simulink model "rocket_upwork"  (R2026a)
settings: Solver=ode15s  StopTime=150  FixedStep=1/3000  MaxStep=0.001  RelTol=1e-6
InitFcn:
  | matl;
undefined symbols (not defined in the file or in its folder): rocket
libraries: aerolibasang x2, simulink x1, aerolibfltsims x1, aerolibatmos2 x1, aerolibadyn x1
settings Model: Creator=evilcatzilla  LastModifiedBy=carlos
settings SolverCC: MaxConsecutiveMinStep=10  SolverResetMethod=Robust
settings SimscapeCC: SimscapeLogDataHistory=5000  SimscapeLogType=none  SimscapeNominalValues="[{\"value\":\"1\",\"unit\":\"A\"},{\"value\":\"1\",\"unit\":\"bar\"},{\"value\":\"1\",\"unit\":\"cm^2\"},{\"value\":\"1\",\"unit\":\"cm^3/s\"},{\"value\":\"1\",\"unit\":\"kJ/kg\"},{\"value\":\"1\",\"unit\":\"kW\"},{\"value\":\"1\",\"unit\":\"l\"},{\"value\":\"1\",\"unit\":\"N\"},{\"value\":\"1\",\"unit\":\"N*m\"},{\"value\":\"1\",\"unit\":\"V\"}]"  SimscapeLogDecimation=1

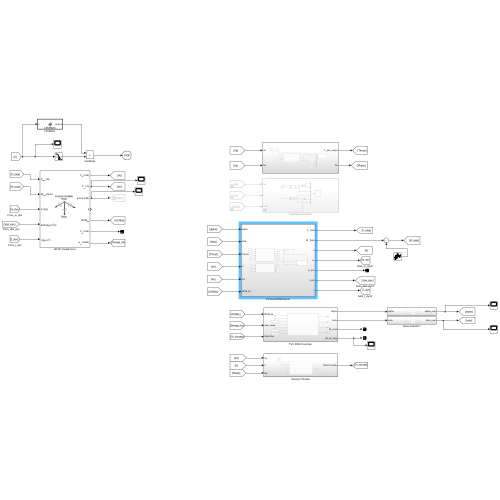
[thumbnail: Simulink's stored preview of the top-level diagram]
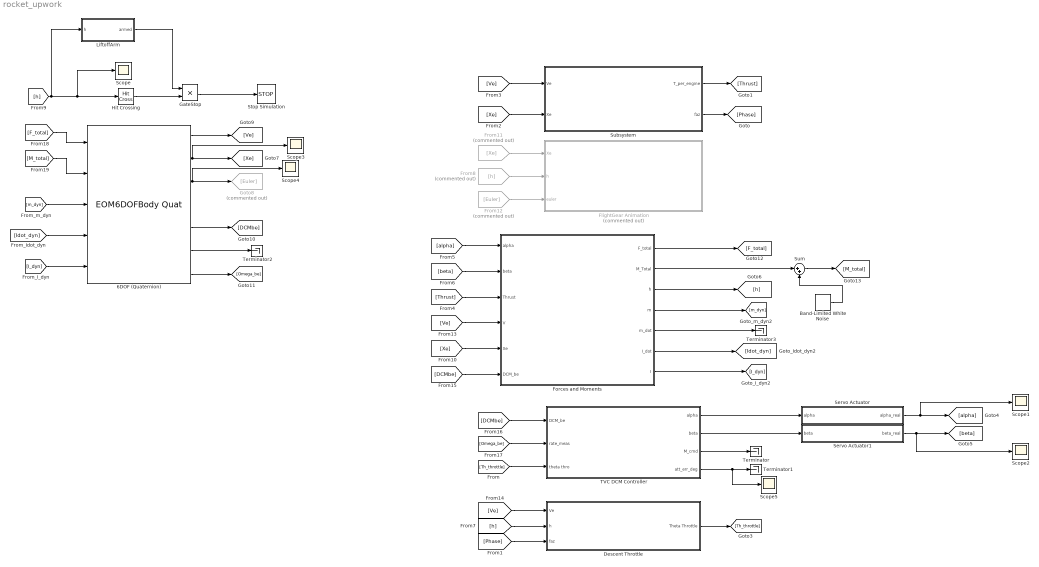
== system rocket_upwork ==
  6DOF (Quaternion) : EOM6DOFBodyQuat  mtype=Custom Variable  eul_0=[0 deg2rad(85) 0]  mass_0=rocket.m0_computed  mass_f=2.0  inertia=diag([rocket.Ixx, rocket.Iyy, rocket.Izz])
  Band-Limited White Noise : simulink/Sources/Band-Limited White Noise  Cov=4e-6  Ts=0.01  seed=[23341 23342 23343]
  Descent Throttle : Subsystem
  FlightGear Animation : Subsystem  Commented=on
  Forces and Moments : Subsystem
  From11 : From  Commented=on  GotoTag=Xe
  From12 : From  Commented=on  GotoTag=Euler
  From8 : From  Commented=on  GotoTag=h
  GateStop : Product
  Goto8 : Goto  Commented=on  GotoTag=Euler
  Hit Crossing : HitCross  HitCrossingDirection=falling
  LiftoffArm : MATLAB Function  TreatAsAtomicUnit=on  SystemSampleTime=0.001
  Scope{,1..5} (6 alike) : Scope
      Scope settings: ActiveDisplayYMinimum=-1.94208  ActiveDisplayYMaximum=17.47869
      Scope1 settings: ActiveDisplayYMinimum=-0.94567  ActiveDisplayYMaximum=1.34881  DataLoggingVariableName=ScopeData2
      Scope2 settings: ActiveDisplayYMinimum=-1.10174  ActiveDisplayYMaximum=1.06476  DataLoggingVariableName=ScopeData3
      Scope3 settings: ActiveDisplayYMinimum=-25.2743  ActiveDisplayYMaximum=72.10268  DataLoggingVariableName=ScopeData4
      Scope4 settings: ActiveDisplayYMinimum=-3.9266  ActiveDisplayYMaximum=3.92558  DataLoggingVariableName=ScopeData5
      Scope5 settings: ActiveDisplayYMinimum=-20.36974  ActiveDisplayYMaximum=7.70273  DataLoggingVariableName=ScopeData7
  Servo Actuator : Subsystem
  Servo Actuator1 : Subsystem
  Stop Simulation : Stop
  Subsystem : Subsystem
  Sum : Sum  Inputs=|++
  TVC DCM Controller : Subsystem
  Terminator{,1..3} (4 alike) : Terminator
  wires:
  TVC DCM Controller/3(M_cmd) -> Terminator/1
  TVC DCM Controller/4(att_err_deg) -> Terminator1/1, Scope5/1
  [h] -> Descent Throttle/2(h)
  From8/1 -> FlightGear Animation/2(h)
  From11/1 -> FlightGear Animation/1(Xe)
  From12/1 -> FlightGear Animation/3(euler)
  [Ve] -> Descent Throttle/1(Ve)
  [DCMbe] -> TVC DCM Controller/1(DCM_be)
  [Omega_be] -> TVC DCM Controller/2(rate_meas)
  Band-Limited White Noise/1 -> Sum/2
  Sum/1 -> [M_total]
  TVC DCM Controller/1(alpha) -> Servo Actuator/1(alpha)
  Servo Actuator/1(alpha_real) -> [alpha], Scope1/1
  TVC DCM Controller/2(beta) -> Servo Actuator1/1(beta)
  Servo Actuator1/1(beta_real) -> [beta], Scope2/1
  Descent Throttle/1(Theta Throttle) -> [Th_throttle]
  [Th_throttle] -> TVC DCM Controller/3(theta thro)
  [Phase] -> Descent Throttle/3(faz)
  Subsystem/2(faz) -> [Phase]
  Subsystem/1(T_per_engine) -> [Thrust]
  [Xe] -> Subsystem/2(Xe)
  [Ve] -> Subsystem/1(Ve)
  [I_dyn] -> 6DOF (Quaternion)/5
  [Idot_dyn] -> 6DOF (Quaternion)/4
  [m_dyn] -> 6DOF (Quaternion)/3
  [F_total] -> 6DOF (Quaternion)/1
  [M_total] -> 6DOF (Quaternion)/2
  [h] -> Scope/1, Hit Crossing/1, LiftoffArm/1(h)
  Forces and Moments/7(I) -> [I_dyn]
  Forces and Moments/6(I_dot) -> [Idot_dyn]
  Forces and Moments/5(m_dot) -> Terminator3/1
  Forces and Moments/4(m) -> [m_dyn]
  [Thrust] -> Forces and Moments/3(Thrust)
  Forces and Moments/2(M_Total) -> Sum/1
  Forces and Moments/3(h) -> [h]
  Forces and Moments/1(F_total) -> [F_total]
  [DCMbe] -> Forces and Moments/6(DCM_be)
  [Xe] -> Forces and Moments/5(Xe)
  [Ve] -> Forces and Moments/4(V)
  [beta] -> Forces and Moments/2(beta)
  [alpha] -> Forces and Moments/1(alpha)
  6DOF (Quaternion)/1 -> [Ve]
  6DOF (Quaternion)/2 -> Scope3/1, [Xe]
  6DOF (Quaternion)/3 -> Scope4/1, Goto8/1
  6DOF (Quaternion)/5 -> [DCMbe]
  6DOF (Quaternion)/6 -> Terminator2/1
  6DOF (Quaternion)/7 -> [Omega_be]
  GateStop/1 -> Stop Simulation/1
  LiftoffArm/1(armed) -> GateStop/1
  Hit Crossing/1 -> GateStop/2

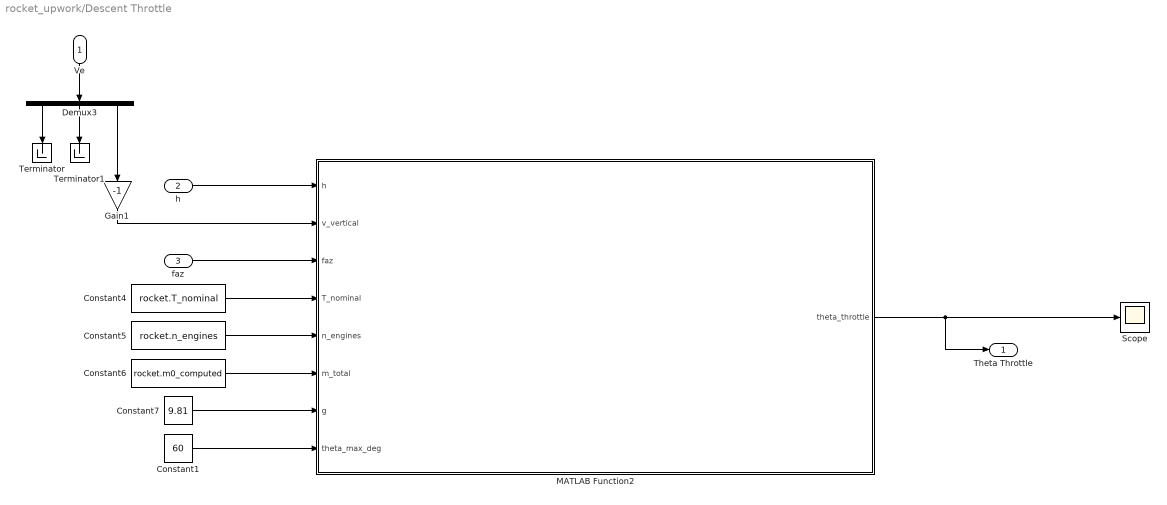
== system rocket_upwork/Descent Throttle ==
  Ve : Inport
  h : Inport  Port=2
  faz : Inport  Port=3
  Constant1 : Constant  Value=60
  Constant4 : Constant  Value=rocket.T_nominal
  Constant5 : Constant  Value=rocket.n_engines
  Constant6 : Constant  Value=rocket.m0_computed
  Constant7 : Constant  Value=9.81
  Demux3 : Demux  Outputs=3
  Gain1 : Gain  Gain=-1
  MATLAB Function2 : MATLAB Function  TreatAsAtomicUnit=on
  Scope : Scope
      settings: ActiveDisplayYMinimum=-0.1309  ActiveDisplayYMaximum=1.1781  DataLoggingVariableName=ScopeData6
  Terminator : Terminator
  Terminator1 : Terminator
  Theta Throttle : Outport
  wires:
  Ve/1 -> Demux3/1
  Demux3/3 -> Gain1/1
  Demux3/2 -> Terminator1/1
  Demux3/1 -> Terminator/1
  h/1 -> MATLAB Function2/1(h)
  Gain1/1 -> MATLAB Function2/2(v_vertical)
  Constant7/1 -> MATLAB Function2/7(g)
  Constant5/1 -> MATLAB Function2/5(n_engines)
  Constant6/1 -> MATLAB Function2/6(m_total)
  Constant4/1 -> MATLAB Function2/4(T_nominal)
  MATLAB Function2/1(theta_throttle) -> Theta Throttle/1, Scope/1
  faz/1 -> MATLAB Function2/3(faz)
  Constant1/1 -> MATLAB Function2/8(theta_max_deg)

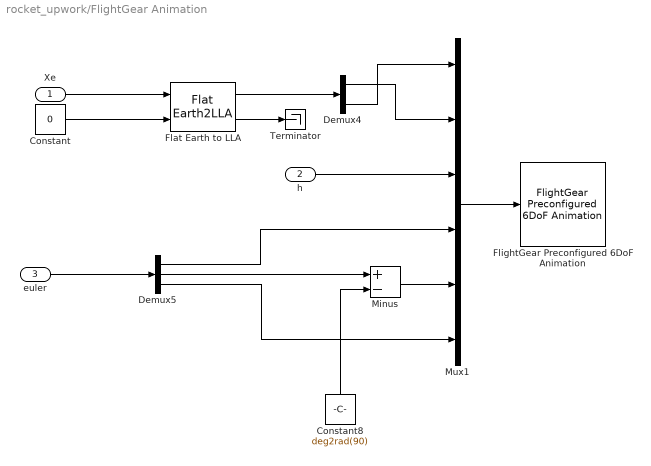
== system rocket_upwork/FlightGear Animation ==
  Xe : Inport
  h : Inport  Port=2
  euler : Inport  Port=3
  Constant : Constant  Value=0
  Constant8 : Constant  Value=deg2rad(90)
  Demux4 : Demux  Outputs=2
  Demux5 : Demux  Outputs=3
  Flat Earth to LLA : FlatEarth2LLA  R=6378137  LL0=[37.61889 -122.37500]
  FlightGear Preconfigured 6DoF Animation : aerolibfltsims/FlightGear Preconfigured 6DoF Animation  xFlightGearVersion=v2019.1  DestinationIpAddress=127.0.0.1  DestinationPort=5502  SampleTime=1/30  packetVersion=24
  Minus : Sum  Inputs=+-
  Mux1 : Mux  Inputs=6
  Terminator : Terminator
  wires:
  Constant/1 -> Flat Earth to LLA/2
  Demux4/1 -> Mux1/2
  Constant8/1 -> Minus/2
  Demux5/2 -> Minus/1
  Minus/1 -> Mux1/5
  Demux5/1 -> Mux1/4
  Demux5/3 -> Mux1/6
  Mux1/1 -> FlightGear Preconfigured 6DoF Animation/1
  Demux4/2 -> Mux1/1
  Flat Earth to LLA/1 -> Demux4/1
  Flat Earth to LLA/2 -> Terminator/1
  euler/1 -> Demux5/1
  h/1 -> Mux1/3
  Xe/1 -> Flat Earth to LLA/1

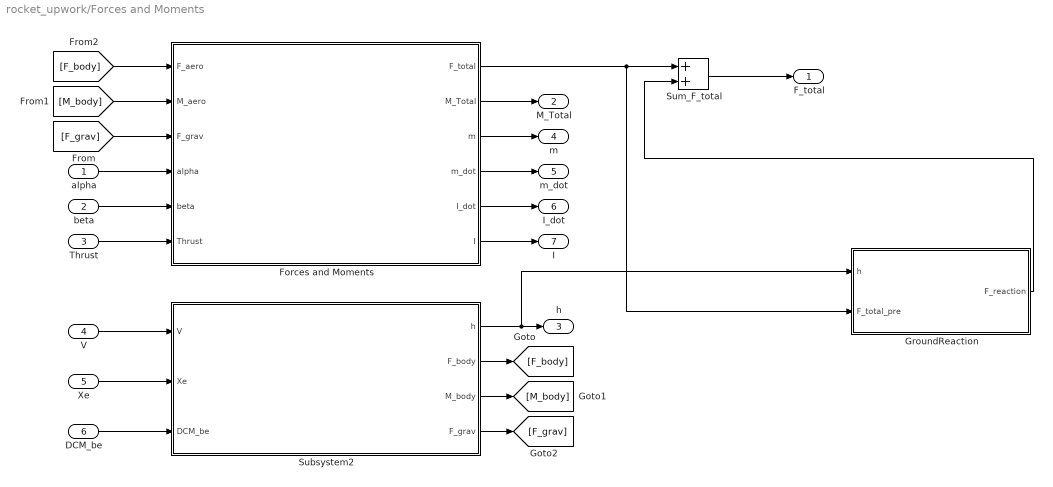
== system rocket_upwork/Forces and Moments ==
  alpha : Inport
  beta : Inport  Port=2
  Thrust : Inport  Port=3
  V : Inport  Port=4
  Xe : Inport  Port=5
  DCM_be : Inport  Port=6
  Forces and Moments : Subsystem
  GroundReaction : MATLAB Function  TreatAsAtomicUnit=on
  Subsystem2 : Subsystem
  Sum_F_total : Sum
  F_total : Outport
  M_Total : Outport  Port=2
  h : Outport  Port=3
  m : Outport  Port=4
  m_dot : Outport  Port=5
  I_dot : Outport  Port=6
  I : Outport  Port=7
  wires:
  alpha/1 -> Forces and Moments/4(alpha)
  DCM_be/1 -> Subsystem2/3(DCM_be)
  Xe/1 -> Subsystem2/2(Xe)
  beta/1 -> Forces and Moments/5(beta)
  Thrust/1 -> Forces and Moments/6(Thrust)
  Forces and Moments/2(M_Total) -> M_Total/1
  Subsystem2/1(h) -> GroundReaction/1(h), h/1
  V/1 -> Subsystem2/1(V)
  [F_grav] -> Forces and Moments/3(F_grav)
  [M_body] -> Forces and Moments/2(M_aero)
  [F_body] -> Forces and Moments/1(F_aero)
  Subsystem2/2(F_body) -> [F_body]
  Subsystem2/4(F_grav) -> [F_grav]
  Subsystem2/3(M_body) -> [M_body]
  Forces and Moments/6(I) -> I/1
  Forces and Moments/5(I_dot) -> I_dot/1
  Forces and Moments/4(m_dot) -> m_dot/1
  Forces and Moments/3(m) -> m/1
  Forces and Moments/1(F_total) -> GroundReaction/2(F_total_pre), Sum_F_total/1
  GroundReaction/1(F_reaction) -> Sum_F_total/2
  Sum_F_total/1 -> F_total/1

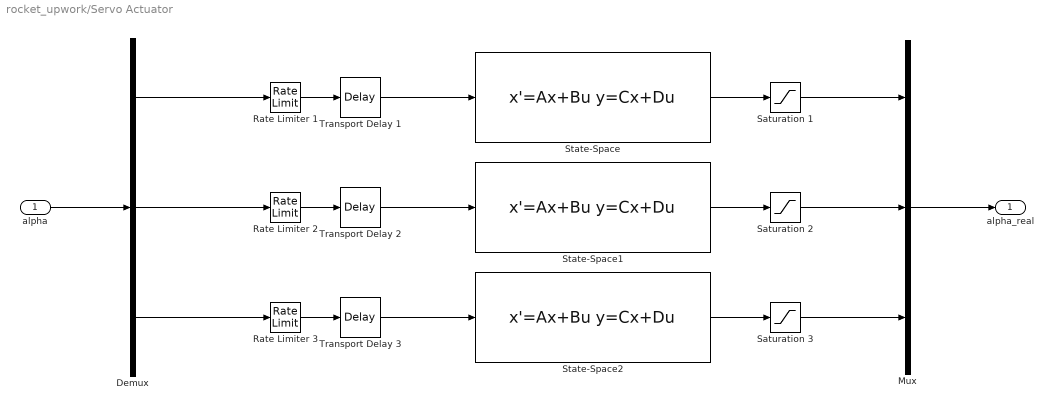
== system rocket_upwork/Servo Actuator ==
  alpha : Inport
  Demux : Demux  Outputs=3
  Mux : Mux  Inputs=3
  Rate Limiter 1 : RateLimiter  RisingSlewLimit=deg2rad(rocket.servo.max_rate_dps)  FallingSlewLimit=-deg2rad(rocket.servo.max_rate_dps)  SampleTimeMode=inherited
  Rate Limiter 2 : RateLimiter  RisingSlewLimit=deg2rad(rocket.servo.max_rate_dps)  FallingSlewLimit=-deg2rad(rocket.servo.max_rate_dps)  SampleTimeMode=inherited
  Rate Limiter 3 : RateLimiter  RisingSlewLimit=deg2rad(rocket.servo.max_rate_dps)  FallingSlewLimit=-deg2rad(rocket.servo.max_rate_dps)  SampleTimeMode=inherited
  Saturation 1 : Saturate  UpperLimit=deg2rad(75)  LowerLimit=deg2rad(-75)
  Saturation 2 : Saturate  UpperLimit=deg2rad(75)  LowerLimit=deg2rad(-75)
  Saturation 3 : Saturate  UpperLimit=deg2rad(75)  LowerLimit=deg2rad(-75)
  State-Space : StateSpace  A="[0  1; -rocket.servo.wn^2  -2*rocket.servo.zeta*rocket.servo.wn]"  B=[0; rocket.servo.wn^2]  C="[1  0]"  D=0  InitialCondition=[0;0]
  State-Space1 : StateSpace  A="[0  1; -rocket.servo.wn^2  -2*rocket.servo.zeta*rocket.servo.wn]"  B=[0; rocket.servo.wn^2]  C="[1  0]"  D=0  InitialCondition=[0;0]
  State-Space2 : StateSpace  A="[0  1; -rocket.servo.wn^2  -2*rocket.servo.zeta*rocket.servo.wn]"  B=[0; rocket.servo.wn^2]  C="[1  0]"  D=0  InitialCondition=[0;0]
  Transport Delay 1 : TransportDelay  DelayTime=rocket.servo.delay_s
  Transport Delay 2 : TransportDelay  DelayTime=rocket.servo.delay_s
  Transport Delay 3 : TransportDelay  DelayTime=rocket.servo.delay_s
  alpha_real : Outport
  wires:
  Rate Limiter 1/1 -> Transport Delay 1/1
  State-Space/1 -> Saturation 1/1
  Transport Delay 1/1 -> State-Space/1
  alpha/1 -> Demux/1
  Transport Delay 2/1 -> State-Space1/1
  State-Space1/1 -> Saturation 2/1
  Rate Limiter 2/1 -> Transport Delay 2/1
  Rate Limiter 3/1 -> Transport Delay 3/1
  State-Space2/1 -> Saturation 3/1
  Transport Delay 3/1 -> State-Space2/1
  Demux/3 -> Rate Limiter 3/1
  Demux/2 -> Rate Limiter 2/1
  Demux/1 -> Rate Limiter 1/1
  Saturation 1/1 -> Mux/1
  Saturation 2/1 -> Mux/2
  Saturation 3/1 -> Mux/3
  Mux/1 -> alpha_real/1

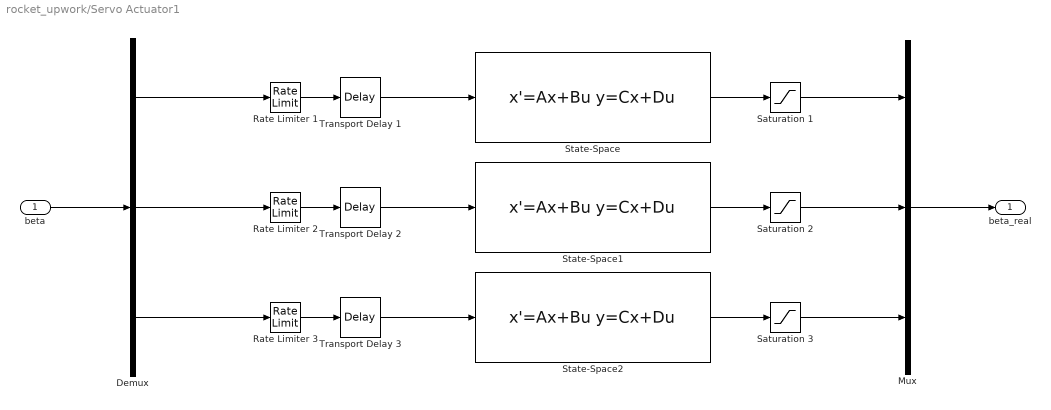
== system rocket_upwork/Servo Actuator1 ==
  beta : Inport
  Demux : Demux  Outputs=3
  Mux : Mux  Inputs=3
  Rate Limiter 1 : RateLimiter  RisingSlewLimit=deg2rad(rocket.servo.max_rate_dps)  FallingSlewLimit=-deg2rad(rocket.servo.max_rate_dps)  SampleTimeMode=inherited
  Rate Limiter 2 : RateLimiter  RisingSlewLimit=deg2rad(rocket.servo.max_rate_dps)  FallingSlewLimit=-deg2rad(rocket.servo.max_rate_dps)  SampleTimeMode=inherited
  Rate Limiter 3 : RateLimiter  RisingSlewLimit=deg2rad(rocket.servo.max_rate_dps)  FallingSlewLimit=-deg2rad(rocket.servo.max_rate_dps)  SampleTimeMode=inherited
  Saturation 1 : Saturate  UpperLimit=deg2rad(75)  LowerLimit=deg2rad(-75)
  Saturation 2 : Saturate  UpperLimit=deg2rad(75)  LowerLimit=deg2rad(-75)
  Saturation 3 : Saturate  UpperLimit=deg2rad(75)  LowerLimit=deg2rad(-75)
  State-Space : StateSpace  A="[0  1; -rocket.servo.wn^2  -2*rocket.servo.zeta*rocket.servo.wn]"  B=[0; rocket.servo.wn^2]  C="[1  0]"  D=0  InitialCondition=[0;0]
  State-Space1 : StateSpace  A="[0  1; -rocket.servo.wn^2  -2*rocket.servo.zeta*rocket.servo.wn]"  B=[0; rocket.servo.wn^2]  C="[1  0]"  D=0  InitialCondition=[0;0]
  State-Space2 : StateSpace  A="[0  1; -rocket.servo.wn^2  -2*rocket.servo.zeta*rocket.servo.wn]"  B=[0; rocket.servo.wn^2]  C="[1  0]"  D=0  InitialCondition=[0;0]
  Transport Delay 1 : TransportDelay  DelayTime=rocket.servo.delay_s
  Transport Delay 2 : TransportDelay  DelayTime=rocket.servo.delay_s
  Transport Delay 3 : TransportDelay  DelayTime=rocket.servo.delay_s
  beta_real : Outport
  wires:
  Saturation 2/1 -> Mux/2
  beta/1 -> Demux/1
  State-Space1/1 -> Saturation 2/1
  Transport Delay 2/1 -> State-Space1/1
  Saturation 1/1 -> Mux/1
  Saturation 3/1 -> Mux/3
  Mux/1 -> beta_real/1
  Rate Limiter 2/1 -> Transport Delay 2/1
  Transport Delay 1/1 -> State-Space/1
  Demux/3 -> Rate Limiter 3/1
  Demux/1 -> Rate Limiter 1/1
  Demux/2 -> Rate Limiter 2/1
  Rate Limiter 3/1 -> Transport Delay 3/1
  State-Space2/1 -> Saturation 3/1
  Transport Delay 3/1 -> State-Space2/1
  State-Space/1 -> Saturation 1/1
  Rate Limiter 1/1 -> Transport Delay 1/1

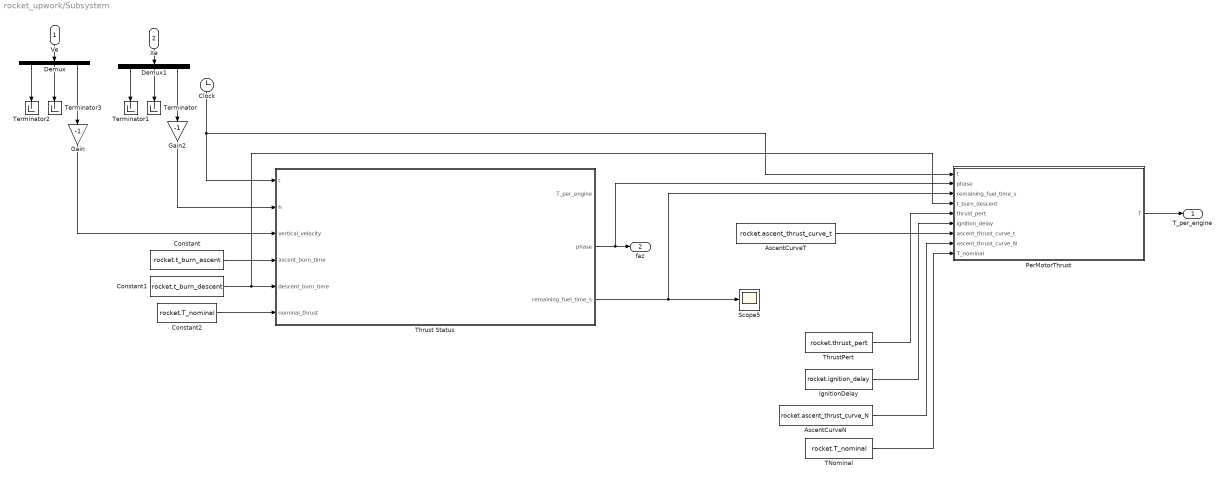
== system rocket_upwork/Subsystem ==
  Ve : Inport
  Xe : Inport  Port=2
  AscentCurveN : Constant  Value=rocket.ascent_thrust_curve_N
  AscentCurveT : Constant  Value=rocket.ascent_thrust_curve_t
  Clock : Clock
  Constant : Constant  Value=rocket.t_burn_ascent
  Constant1 : Constant  Value=rocket.t_burn_descent
  Constant2 : Constant  Value=rocket.T_nominal
  Demux : Demux  Outputs=3
  Demux1 : Demux  Outputs=3
  Gain : Gain  Gain=-1
  Gain2 : Gain  Gain=-1
  IgnitionDelay : Constant  Value=rocket.ignition_delay
  PerMotorThrust : MATLAB Function  TreatAsAtomicUnit=on
  Scope5 : Scope
      settings: ActiveDisplayYMinimum=-1.25  ActiveDisplayYMaximum=11.25
  TNominal : Constant  Value=rocket.T_nominal
  Terminator{,1..3} (4 alike) : Terminator
  Thrust Status : MATLAB Function  TreatAsAtomicUnit=on
  ThrustPert : Constant  Value=rocket.thrust_pert
  T_per_engine : Outport
  faz : Outport  Port=2
  wires:
  Ve/1 -> Demux/1
  Xe/1 -> Demux1/1
  Demux/2 -> Terminator3/1
  Thrust Status/2(phase) -> faz/1, PerMotorThrust/2(phase)
  Demux1/3 -> Gain2/1
  Demux1/1 -> Terminator1/1
  Demux/3 -> Gain/1
  Thrust Status/3(remaining_fuel_time_s) -> Scope5/1, PerMotorThrust/3(remaining_fuel_time_s)
  Gain2/1 -> Thrust Status/2(h)
  Demux/1 -> Terminator2/1
  Demux1/2 -> Terminator/1
  Clock/1 -> Thrust Status/1(t), PerMotorThrust/1(t)
  Gain/1 -> Thrust Status/3(vertical_velocity)
  Constant/1 -> Thrust Status/4(ascent_burn_time)
  Constant1/1 -> Thrust Status/5(descent_burn_time), PerMotorThrust/4(t_burn_descent)
  Constant2/1 -> Thrust Status/6(nominal_thrust)
  ThrustPert/1 -> PerMotorThrust/5(thrust_pert)
  IgnitionDelay/1 -> PerMotorThrust/6(ignition_delay)
  AscentCurveT/1 -> PerMotorThrust/7(ascent_thrust_curve_t)
  AscentCurveN/1 -> PerMotorThrust/8(ascent_thrust_curve_N)
  TNominal/1 -> PerMotorThrust/9(T_nominal)
  PerMotorThrust/1(T) -> T_per_engine/1

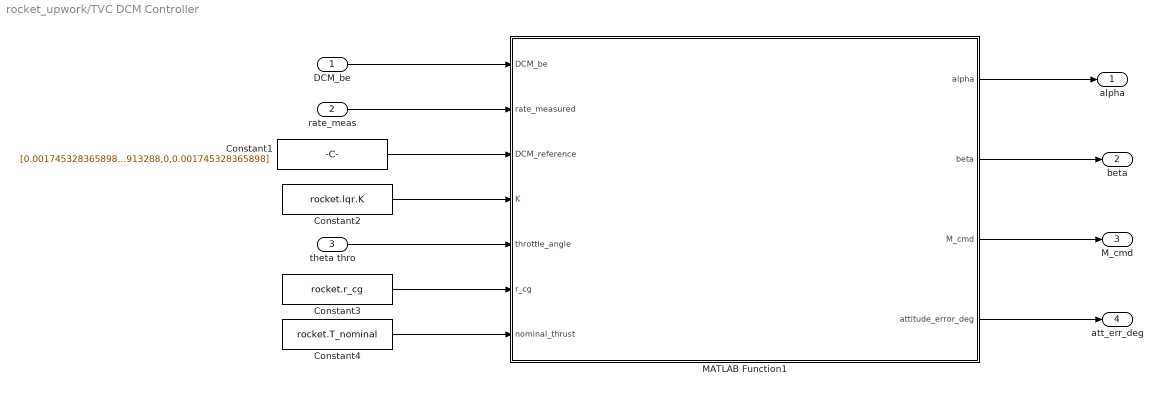
== system rocket_upwork/TVC DCM Controller ==
  DCM_be : Inport
  rate_meas : Inport  Port=2
  theta thro : Inport  Port=3
  Constant1 : Constant  Value=[0.001745328365898,0,-0.999998476913288;0,1,0;0.999998476913288,0,0.001745328365898]
  Constant2 : Constant  Value=rocket.lqr.K
  Constant3 : Constant  Value=rocket.r_cg
  Constant4 : Constant  Value=rocket.T_nominal
  MATLAB Function1 : MATLAB Function  TreatAsAtomicUnit=on
  alpha : Outport
  beta : Outport  Port=2
  M_cmd : Outport  Port=3
  att_err_deg : Outport  Port=4
  wires:
  Constant2/1 -> MATLAB Function1/4(K)
  rate_meas/1 -> MATLAB Function1/2(rate_measured)
  Constant1/1 -> MATLAB Function1/3(DCM_reference)
  MATLAB Function1/1(alpha) -> alpha/1
  DCM_be/1 -> MATLAB Function1/1(DCM_be)
  MATLAB Function1/2(beta) -> beta/1
  MATLAB Function1/3(M_cmd) -> M_cmd/1
  MATLAB Function1/4(attitude_error_deg) -> att_err_deg/1
  Constant3/1 -> MATLAB Function1/6(r_cg)
  Constant4/1 -> MATLAB Function1/7(nominal_thrust)
  theta thro/1 -> MATLAB Function1/5(throttle_angle)

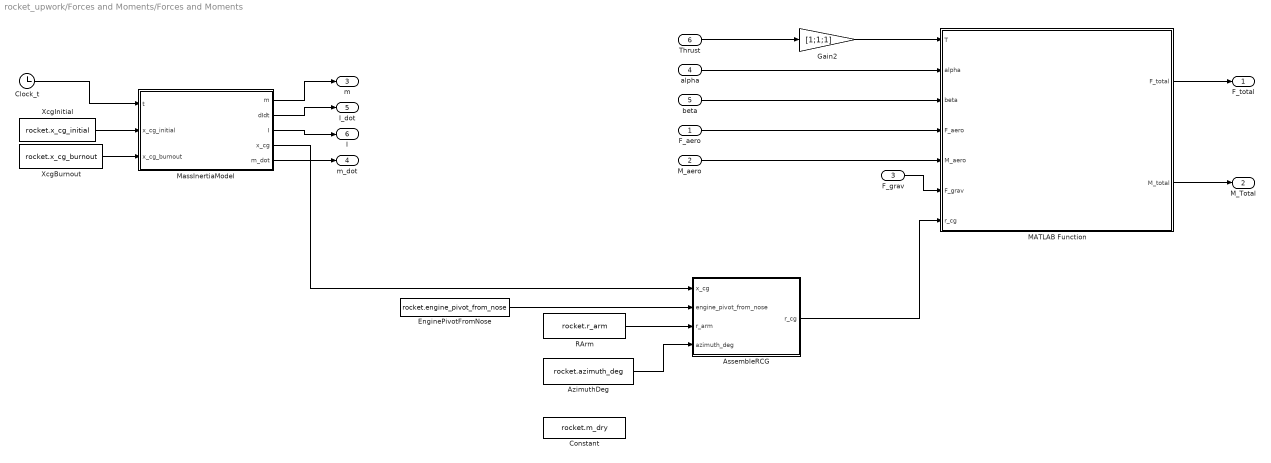
== system rocket_upwork/Forces and Moments/Forces and Moments ==
  F_aero : Inport
  M_aero : Inport  Port=2
  F_grav : Inport  Port=3
  alpha : Inport  Port=4
  beta : Inport  Port=5
  Thrust : Inport  Port=6
  AssembleRCG : MATLAB Function  TreatAsAtomicUnit=on
  AzimuthDeg : Constant  Value=rocket.azimuth_deg
  Clock_t : Clock
  Constant : Constant  Value=rocket.m_dry
  EnginePivotFromNose : Constant  Value=rocket.engine_pivot_from_nose
  Gain2 : Gain  Gain=[1;1;1]
  MATLAB Function : MATLAB Function  TreatAsAtomicUnit=on
  MassInertiaModel : MATLAB Function  TreatAsAtomicUnit=on
  RArm : Constant  Value=rocket.r_arm
  XcgBurnout : Constant  Value=rocket.x_cg_burnout
  XcgInitial : Constant  Value=rocket.x_cg_initial
  F_total : Outport
  M_Total : Outport  Port=2
  m : Outport  Port=3
  m_dot : Outport  Port=4
  I_dot : Outport  Port=5
  I : Outport  Port=6
  wires:
  Thrust/1 -> Gain2/1
  XcgBurnout/1 -> MassInertiaModel/3(x_cg_burnout)
  XcgInitial/1 -> MassInertiaModel/2(x_cg_initial)
  M_aero/1 -> MATLAB Function/5(M_aero)
  MATLAB Function/1(F_total) -> F_total/1
  Gain2/1 -> MATLAB Function/1(T)
  MATLAB Function/2(M_total) -> M_Total/1
  F_aero/1 -> MATLAB Function/4(F_aero)
  beta/1 -> MATLAB Function/3(beta)
  alpha/1 -> MATLAB Function/2(alpha)
  AssembleRCG/1(r_cg) -> MATLAB Function/7(r_cg)
  MassInertiaModel/4(x_cg) -> AssembleRCG/1(x_cg)
  Clock_t/1 -> MassInertiaModel/1(t)
  F_grav/1 -> MATLAB Function/6(F_grav)
  EnginePivotFromNose/1 -> AssembleRCG/2(engine_pivot_from_nose)
  RArm/1 -> AssembleRCG/3(r_arm)
  AzimuthDeg/1 -> AssembleRCG/4(azimuth_deg)
  MassInertiaModel/3(I) -> I/1
  MassInertiaModel/2(dIdt) -> I_dot/1
  MassInertiaModel/5(m_dot) -> m_dot/1
  MassInertiaModel/1(m) -> m/1

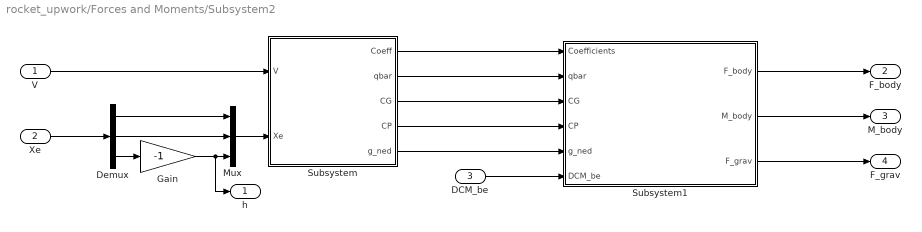
== system rocket_upwork/Forces and Moments/Subsystem2 ==
  V : Inport
  Xe : Inport  Port=2
  DCM_be : Inport  Port=3
  Demux : Demux  Outputs=3
  Gain : Gain  Gain=-1
  Mux : Mux  Inputs=3
  Subsystem : Subsystem
  Subsystem1 : Subsystem
  h : Outport
  F_body : Outport  Port=2
  M_body : Outport  Port=3
  F_grav : Outport  Port=4
  wires:
  Subsystem/1(Coeff) -> Subsystem1/1(Coefficients)
  Demux/1 -> Mux/1
  Demux/3 -> Gain/1
  Subsystem/3(CG) -> Subsystem1/3(CG)
  Subsystem/4(CP) -> Subsystem1/4(CP)
  Subsystem/2(qbar) -> Subsystem1/2(qbar)
  Demux/2 -> Mux/2
  Mux/1 -> Subsystem/2(Xe)
  Subsystem1/2(M_body) -> M_body/1
  Subsystem/5(g_ned) -> Subsystem1/5(g_ned)
  DCM_be/1 -> Subsystem1/6(DCM_be)
  Xe/1 -> Demux/1
  Gain/1 -> Mux/3, h/1
  V/1 -> Subsystem/1(V)
  Subsystem1/1(F_body) -> F_body/1
  Subsystem1/3(F_grav) -> F_grav/1

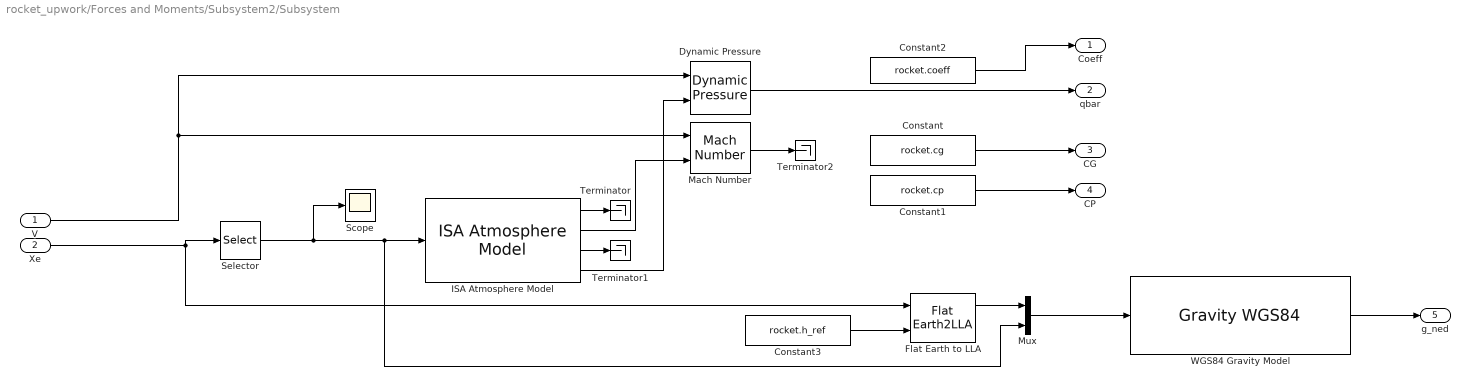
== system rocket_upwork/Forces and Moments/Subsystem2/Subsystem ==
  V : Inport
  Xe : Inport  Port=2
  Constant : Constant  Value=rocket.cg
  Constant1 : Constant  Value=rocket.cp
  Constant2 : Constant  Value=rocket.coeff
  Constant3 : Constant  Value=rocket.h_ref
  Dynamic Pressure : aerolibasang/Dynamic Pressure
  Flat Earth to LLA : FlatEarth2LLA  R=6378137
  ISA Atmosphere Model : aerolibatmos2/ISA Atmosphere Model  useExtended=off  action=Warning  custom=off  viscosityOut=off  g=9.80665  gamma=1.4  R=287.0531  L=0.0065  h_trop=11000  h_strat=20000  rho0=1.225  P0=101325  T0=288.15  h0=0  S=110.4  Tref=273.15  muref=1.716e-5
  Mach Number : aerolibasang/Mach Number
  Mux : Mux  Inputs=2
  Scope : Scope
      settings: ActiveDisplayYMinimum=-14.46754  ActiveDisplayYMaximum=130.20784  DataLoggingVariableName=ScopeData6
  Selector : Selector  InputPortWidth=3  IndexOptions=Index vector (dialog)  Indices=3  OutputSizes=1
  Terminator : Terminator
  Terminator1 : Terminator
  Terminator2 : Terminator
  "WGS84 Gravity Model  " : GravityWGS84
  Coeff : Outport
  qbar : Outport  Port=2
  CG : Outport  Port=3
  CP : Outport  Port=4
  g_ned : Outport  Port=5
  wires:
  V/1 -> Mach Number/1, Dynamic Pressure/1
  Mach Number/1 -> Terminator2/1
  ISA Atmosphere Model/1 -> Terminator/1
  ISA Atmosphere Model/3 -> Terminator1/1
  Xe/1 -> Selector/1, Flat Earth to LLA/1
  ISA Atmosphere Model/4 -> Dynamic Pressure/2
  ISA Atmosphere Model/2 -> Mach Number/2
  Selector/1 -> Scope/1, Mux/2, ISA Atmosphere Model/1
  Mux/1 -> "WGS84 Gravity Model  "/1
  Flat Earth to LLA/1 -> Mux/1
  Constant3/1 -> Flat Earth to LLA/2
  "WGS84 Gravity Model  "/1 -> g_ned/1
  Dynamic Pressure/1 -> qbar/1
  Constant1/1 -> CP/1
  Constant2/1 -> Coeff/1
  Constant/1 -> CG/1

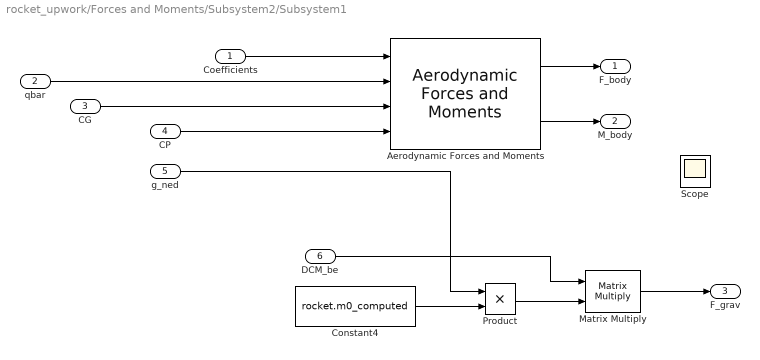
== system rocket_upwork/Forces and Moments/Subsystem2/Subsystem1 ==
  Coefficients : Inport
  qbar : Inport  Port=2
  CG : Inport  Port=3
  CP : Inport  Port=4
  g_ned : Inport  Port=5
  DCM_be : Inport  Port=6
  "Aerodynamic Forces and Moments " : aerolibadyn/Aerodynamic Forces and Moments   inputAxes=Body  outputForceAxes=Body  outputMomentAxes=Body  S=0.0854  b=0.0742  cbar=1.15
  Constant4 : Constant  Value=rocket.m0_computed
  Matrix Multiply : Product  Multiplication=Matrix(*)
  Product : Product
  Scope : Scope
      settings: ActiveDisplayYMinimum=-1  ActiveDisplayYMaximum=1  DataLoggingVariableName=ScopeData4
  F_body : Outport
  M_body : Outport  Port=2
  F_grav : Outport  Port=3
  wires:
  g_ned/1 -> Product/1
  qbar/1 -> "Aerodynamic Forces and Moments "/2
  Coefficients/1 -> "Aerodynamic Forces and Moments "/1
  "Aerodynamic Forces and Moments "/1 -> F_body/1
  Matrix Multiply/1 -> F_grav/1
  CG/1 -> "Aerodynamic Forces and Moments "/3
  "Aerodynamic Forces and Moments "/2 -> M_body/1
  Constant4/1 -> Product/2
  DCM_be/1 -> Matrix Multiply/1
  CP/1 -> "Aerodynamic Forces and Moments "/4
  Product/1 -> Matrix Multiply/2

== matlab function rocket_upwork/Subsystem/PerMotorThrust ==
  data: t input; T output; phase input; remaining_fuel_time_s input; t_burn_descent input; thrust_pert input; ignition_delay input; ascent_thrust_curve_t input; ascent_thrust_curve_N input; T_nominal input
function T = PerMotorThrust(t, phase, remaining_fuel_time_s, t_burn_descent, ...
    thrust_pert, ignition_delay, ascent_thrust_curve_t, ascent_thrust_curve_N, T_nominal)
% Per-motor thrust: ascent motors follow the real static-test thrust curve
% (raw scale reading, see rocket.ascent_thrust_curve_* comments in matl.m for
% the mass-loss-correction caveat); descent motors keep the flat T_nominal
% placeholder, unchanged from before this task. Both phases support a
% per-motor thrust_pert (fractional multiplier) and ignition_delay (s) for
% sensitivity studies, zero by default (symmetric baseline).
%
% time_in_phase is derived here rather than passed in, because
% remaining_fuel_time_s only counts down meaningfully during phase 3
% (descent burn) - during phase 1 (ascent) it is just a constant equal to
% descent_burn_time (see Thrust Status chart), not usable for ascent
% timing. Ascent phase starts at simulation t=0 by construction (Thrust
% Status initializes to phase 1 on its very first evaluation), so t itself
% is the correct time-in-phase for ascent.

T = zeros(3, 1);

if phase == 1
    time_in_phase = t;
elseif phase == 3
    time_in_phase = t_burn_descent - remaining_fuel_time_s;
else
    time_in_phase = -1; % forces t_local < 0 below, T stays 0
end

t_curve_end = ascent_thrust_curve_t(end);

for i = 1:3
    t_local = time_in_phase - ignition_delay(i);

    if phase == 1 && t_local >= 0
        t_clamped = min(t_local, t_curve_end);
        T_base = interp1(ascent_thrust_curve_t, ascent_thrust_curve_N, ...
            t_clamped, 'linear', 'extrap');
        T(i) = T_base * (1 + thrust_pert(i));
    elseif phase == 3 && t_local >= 0
        T(i) = T_nominal * (1 + thrust_pert(i));
    else
        T(i) = 0;
    end
end

end

== matlab function rocket_upwork/Forces and Moments/GroundReaction ==
  data: h input; F_reaction output; F_total_pre input
function F_reaction = GroundReaction(h, F_total_pre)
% Minimal launch-pad ground reaction: holds the vehicle at h<=0 while net
% force on the vertical/thrust axis (body x_b, confirmed via Step 0
% diagnostic - positive x_b opposes gravity at the near-vertical launch
% attitude) is still downward, i.e. thrust has not yet exceeded weight.
% Cancels only the net-downward x_b component exactly (F_total stays
% unchanged once it is net-upward); lateral force (y_b, z_b) and all
% moments are untouched, so TVC attitude correction proceeds normally
% even while grounded. Zero effect once airborne (h > tolerance). This
% is a physics fix (real pad/rail support), not a touchdown-detector
% patch - Hit Crossing/Stop Simulation are untouched.

tol = 0.001;
F_reaction = zeros(3, 1);

if h <= tol
    F_reaction(1) = -min(F_total_pre(1), 0);
end

end

== matlab function rocket_upwork/LiftoffArm ==
  data: h input; armed output
function armed = LiftoffArm(h)
% Latches touchdown detection off during the launch-pad phase, so a
% small residual GroundReaction dip (max observed -0.043m; the
% Hit Crossing block has zero tolerance) cannot be mistaken for a real
% touchdown. PRE_LIFTOFF(0) -> LIFTOFF_CONFIRMED(1) once h exceeds
% 1.0m - about 20x the worst residual dip observed, and ~0.6s after
% real liftoff in the nominal case, comfortably clear of ground-phase
% noise without masking a genuine early-flight problem. Never resets
% back to PRE_LIFTOFF once armed, even if altitude dips again later
% (e.g. a hover phase) - matches Thrust Status's own persistent-state
% style, this project's convention for stateful charts. A fixed
% altitude threshold was deliberately chosen over touching Hit
% Crossing's own tolerance, since the ground-phase dip depth varies
% with thrust_pert/ignition_delay and a tolerance edit would need
% re-justifying for every sweep point.

persistent state
if isempty(state)
    state = int8(0);
end

if state == 0 && h > 1.0
    state = int8(1);
end

armed = double(state);

end

== matlab function rocket_upwork/Descent Throttle/MATLAB Function2 ==
  settings: updateMethod=DISCRETE
  data: theta_throttle output; h input; v_vertical input; faz input; T_nominal input; n_engines input; m_total input; g input; theta_max_deg input
function theta_throttle = descent_tilt_lqr(h, v_vertical, faz, T_nominal, n_engines, m_total, g, theta_max_deg)
    if faz ~= 3
        theta_throttle = 0;
        return;
    end

    T_max_toplam = n_engines * T_nominal;
    theta_max = deg2rad(theta_max_deg);

    theta_hover = acos(min(max(m_total*g/T_max_toplam, -1), 1));

    K_H = -0.2;
    K_V = -0.37986389;

    delta_theta = -(K_H*h + K_V*v_vertical);
    theta_throttle = theta_hover + delta_theta;

    theta_throttle = min(max(theta_throttle, 0), theta_max);

end

== matlab function rocket_upwork/Forces and Moments/Forces and Moments/MATLAB Function ==
  data: T input; F_total output; alpha input; beta input; F_aero input; M_aero input; F_grav input; M_total output; r_cg input
function [F_total, M_total] = rocket_forces_moments(T, alpha, beta, F_aero, M_aero, F_grav, r_cg)

    F_thrust = zeros(3,1);
    M_thrust = zeros(3,1);

    for i = 1:3
        F_i = T(i) * [cos(alpha(i))*cos(beta(i));
                       sin(alpha(i))*cos(beta(i));
                       sin(beta(i))];

        r_i = r_cg(:,i);
        M_i = cross(r_i, F_i);

        F_thrust = F_thrust + F_i;
        M_thrust = M_thrust + M_i;
    end

    F_total = F_thrust + F_aero + F_grav;
    M_total = M_thrust + M_aero;

end

== matlab function rocket_upwork/TVC DCM Controller/MATLAB Function1 ==
  settings: updateMethod=DISCRETE
  data: DCM_be input; alpha output; rate_measured input; DCM_reference input; K input; beta output; M_cmd output; throttle_angle input; attitude_error_deg output; r_cg input; nominal_thrust input
function [alpha, beta, M_cmd, attitude_error_deg] = ...
    tvc_controller_dcm(DCM_be, rate_measured, DCM_reference, ...
                       K, throttle_angle, r_cg, nominal_thrust)

    DCM_be        = reshape(DCM_be,        3, 3);
    DCM_reference = reshape(DCM_reference, 3, 3);
    r_cg          = reshape(r_cg,          3, 3);

    gimbal_limit_rad = deg2rad([-10, 10]);

    gimbal_min = gimbal_limit_rad(1);
    gimbal_max = gimbal_limit_rad(2);

    DCM_error = DCM_be * DCM_reference';

    attitude_error = 0.5 * ...
        [DCM_error(3,2) - DCM_error(2,3);
         DCM_error(1,3) - DCM_error(3,1);
         DCM_error(2,1) - DCM_error(1,2)];

    state_error = [attitude_error;
                   rate_measured];

    M_cmd = -K * state_error;

    attitude_error_deg = rad2deg(attitude_error);

    allocation_matrix = zeros(3,6);

    for i = 1:3
        r_i = r_cg(:,i);

        allocation_matrix(:, 2*i-1) = ...
            cross(r_i, nominal_thrust * [0; 1; 0]);

        allocation_matrix(:, 2*i) = ...
            cross(r_i, nominal_thrust * [0; 0; 1]);
    end

    delta_lqr = pinv(allocation_matrix) * M_cmd;

    max_gimbal_command = max(abs(delta_lqr));

    if max_gimbal_command > gimbal_max
        delta_lqr = delta_lqr * ...
            (gimbal_max / max_gimbal_command);
    end

    alpha = zeros(3,1);
    beta  = zeros(3,1);

    for i = 1:3

        azimuth_angle = atan2(r_cg(3,i), r_cg(2,i));

        alpha_nominal = atan2( ...
            sin(throttle_angle) * cos(azimuth_angle), ...
            cos(throttle_angle));

        beta_nominal = asin( ...
            sin(throttle_angle) * sin(azimuth_angle));

        alpha(i) = alpha_nominal + delta_lqr(2*i-1);
        beta(i)  = beta_nominal  + delta_lqr(2*i);

    end

    overall_gimbal_limit = max( ...
        abs(gimbal_max), ...
        throttle_angle + gimbal_max);

    alpha = min( ...
        max(alpha, -overall_gimbal_limit), ...
        overall_gimbal_limit);

    beta = min( ...
        max(beta, -overall_gimbal_limit), ...
        overall_gimbal_limit);

end

== matlab function rocket_upwork/Subsystem/Thrust Status ==
  settings: updateMethod=DISCRETE
  data: t input; h input; T_per_engine output; vertical_velocity input; ascent_burn_time input; descent_burn_time input; nominal_thrust input; phase output; remaining_fuel_time_s output
function [T_per_engine, phase, remaining_fuel_time_s] = ...
    engine_thrust_status(t, h, vertical_velocity, ...
                        ascent_burn_time, descent_burn_time, nominal_thrust)

    ignition_altitude_m = 15;

    persistent phase_state ignition_time

    if isempty(phase_state)
        phase_state = int8(1);
        ignition_time = 0;
    end

    if phase_state == 1

        if t < ascent_burn_time
            T_per_engine = nominal_thrust;
        else
            phase_state = int8(2);
            T_per_engine = 0;
        end

        remaining_fuel_time_s = descent_burn_time;

    elseif phase_state == 2

        T_per_engine = 0;

        if vertical_velocity < 0 && h <= ignition_altitude_m
            phase_state = int8(3);
            ignition_time = t;
        end

        remaining_fuel_time_s = descent_burn_time;

    else

        elapsed_time = t - ignition_time;

        remaining_fuel_time_s = max( ...
            descent_burn_time - elapsed_time, 0);

        if remaining_fuel_time_s <= 0
            phase_state = int8(4);
            T_per_engine = 0;
        else
            T_per_engine = nominal_thrust;
        end

    end

    phase = double(phase_state);

end

== matlab function rocket_upwork/Forces and Moments/Forces and Moments/MassInertiaModel ==
  data: t input; m output; dIdt output; I output; x_cg output; x_cg_initial input; x_cg_burnout input; m_dot output
function [m, dIdt, I, x_cg, m_dot] = MassInertiaModel(t, x_cg_initial, x_cg_burnout)
% Computes vehicle mass and inertia tensor as propellant burns
% Linear depletion model: mass decreases linearly during burn, then holds constant

%% --- Editable parameters ---
% Reconciled with Kruthick's measured values (mass reconciliation pass):
% m_dry = m_total - m_prop_total = 2000 - 690 = 1310 g. Must stay identical
% to rocket.m_dry in matl.m - see CLAUDE.md known gap on duplicate
% parameter sets.
m_dry    = 1.310;  % kg, mass with no propellant (structure + avionics + empty motors)
m_prop   = 0.690;  % kg, total propellant mass (KNSB), 230 g x 3 motors
t_burn   = 20;     % s, burn duration (must match ThrustMixer)

Ixx_dry  = 0.002;  % kg*m^2, roll-axis inertia (about x_b, nose axis), empty
Iyy_dry  = 0.05;   % kg*m^2, pitch-axis inertia (about y_b), empty
Izz_dry  = 0.05;   % kg*m^2, yaw-axis inertia (about z_b), empty

% How much extra inertia the propellant mass contributes when full
% (rough approximation: propellant sits near the tail, contributes mostly to pitch/yaw)
Ixx_prop = 0.0002;
Iyy_prop = 0.01;
Izz_prop = 0.01;

% x_cg_initial/x_cg_burnout now come in as explicit inputs (not hardcoded
% locals) fed by Constant blocks with Value = rocket.x_cg_initial /
% rocket.x_cg_burnout, same pattern as AssembleRCG's geometry inputs -
% this chart's eML dialect cannot resolve rocket.* struct fields directly.
% See CLAUDE.md known gaps.

%% --- Mass as a function of time ---
if t < t_burn
    frac_burned = t / t_burn;      % 0 at ignition, 1 at burnout
else
    frac_burned = 1;
end

m_remaining_prop = m_prop * (1 - frac_burned);
m = m_dry + m_remaining_prop;

%% --- Mass rate (analytic, matches the piecewise-linear depletion above) ---
if t < t_burn
    m_dot = -m_prop / t_burn;      % negative: mass decreasing while burning
else
    m_dot = 0;
end

%% --- Inertia as a function of remaining propellant ---
Ixx = Ixx_dry + Ixx_prop * (1 - frac_burned);
Iyy = Iyy_dry + Iyy_prop * (1 - frac_burned);
Izz = Izz_dry + Izz_prop * (1 - frac_burned);

I = [Ixx 0 0; 0 Iyy 0; 0 0 Izz];


%% --- dI/dt (derivative of inertia w.r.t. time) ---
if t < t_burn
    dIxx_dt = -Ixx_prop / t_burn;
    dIyy_dt = -Iyy_prop / t_burn;
    dIzz_dt = -Izz_prop / t_burn;
else
    dIxx_dt = 0;
    dIyy_dt = 0;
    dIzz_dt = 0;
end

dIdt = [dIxx_dt 0 0; 0 dIyy_dt 0; 0 0 dIzz_dt];

%% --- Axial CG position as a function of remaining propellant ---
% frac_burned is the propellant mass fraction burned here (equals the time
% fraction because depletion above is linear in time); linear interpolation
% between x_cg_initial and x_cg_burnout is exact for this depletion model.
x_cg = x_cg_initial + (x_cg_burnout - x_cg_initial) * frac_burned;

end

== matlab function rocket_upwork/Forces and Moments/Forces and Moments/AssembleRCG ==
  data: x_cg input; r_cg output; engine_pivot_from_nose input; r_arm input; azimuth_deg input
function r_cg = AssembleRCG(x_cg, engine_pivot_from_nose, r_arm, azimuth_deg)
% Assembles the 3x3 motor moment-arm matrix (columns = motors) fed into
% rocket_forces_moments, with a dynamic axial row driven by x_cg(t).
% Lateral rows (2-3) use the same static per-motor azimuth offset already
% computed in matl.m (rocket.r_arm, rocket.azimuth_deg), unchanged.
% engine_pivot_from_nose/r_arm/azimuth_deg come in as explicit inputs (not
% referenced as rocket.* internally) because this chart's eML dialect does
% not resolve struct-field workspace references inside the function body -
% confirmed empirically (Stateflow:cdr:ErrorsParsingEmlFcn). Same reason
% rocket_forces_moments takes r_cg as an input rather than reading it directly.

r_cg = zeros(3,3);

for i = 1:3
    azimuth_angle = deg2rad(azimuth_deg(i));

    r_cg(1,i) = x_cg - engine_pivot_from_nose;
    r_cg(2,i) = r_arm * cos(azimuth_angle);
    r_cg(3,i) = r_arm * sin(azimuth_angle);
end

end
